simulink library "sm_boom_lift_crawler_lib"  (R2026a)
settings: Solver=VariableStepAuto
undefined symbols (not defined in the file): B, b, base_clr_a, base_clr_d, base_clr_e, base_clr_h, base_clr_s, base_h, base_opc, base_rho, base_t, base_w, F, lines, motion, overlap_l, valves, X, Y, Z
libraries: nesl_utility x155, fl_lib x72, sm_lib x38, SimscapeFluids_lib x18, $bdroot x2, simulink_extras x1, simulink x1, Custom_Valves x1
(part 4 of 4)

== system sm_boom_lift_crawler_lib/Turret Signal ==
  q : Inport
  Bus Creator : BusCreator  Inputs=3
  PS-Simulink Converter1 : nesl_utility/PS-Simulink Converter  PhysicalDomain=network_engine_domain  SubClassName=ps_output  LeftPortType=input  RightPortType=output  PseudoPeriodic=off  Frequencies=[]  VectorFormat=1-D array  Unit=inherit  AffineConversion=off
  PS-Simulink Converter2 : nesl_utility/PS-Simulink Converter  PhysicalDomain=network_engine_domain  SubClassName=ps_output  LeftPortType=input  RightPortType=output  PseudoPeriodic=off  Frequencies=[]  VectorFormat=1-D array  Unit=inherit  AffineConversion=off
  PS-Simulink Converter3 : nesl_utility/PS-Simulink Converter  PhysicalDomain=network_engine_domain  SubClassName=ps_output  LeftPortType=input  RightPortType=output  PseudoPeriodic=off  Frequencies=[]  VectorFormat=1-D array  Unit=inherit  AffineConversion=off
  Revolute Turret : sm_lib/Joints/Revolute Joint  JointMode=Normal  CompositeWrenchDir=FollowerOnBase  CompositeWrenchFrame=BaseFrame  SenseConstraintForce=off  SenseConstraintTorque=off  SenseTotalForce=off  SenseTotalTorque=off  PositionTargetSpecify=on  PositionTargetPriority=High  PositionTargetValue=0  PositionTargetValueUnits=deg  VelocityTargetSpecify=off  VelocityTargetPriority=High  VelocityTargetValue=0  VelocityTargetValueUnits=deg/s  EquilibriumPosition=0  EquilibriumPositionUnits=rad  SpringStiffness=0  SpringStiffnessUnits=N*m/rad  DampingCoefficient=b.r.joint  DampingCoefficientUnits=N*m/(rad/s)  LowerLimitSpecify=off  LowerLimitBound=-90  LowerLimitBoundUnits=deg  LowerLimitStiffness=1e4  LowerLimitStiffnessUnits=N*m/deg  LowerLimitDamping=10  LowerLimitDampingUnits=N*m/(deg/s)  LowerLimitTransitionRegionWidth=0.1  LowerLimitTransitionRegionWidthUnits=deg  UpperLimitSpecify=off  UpperLimitBound=90  UpperLimitBoundUnits=deg  UpperLimitStiffness=1e4  UpperLimitStiffnessUnits=N*m/deg  UpperLimitDamping=10  UpperLimitDampingUnits=N*m/(deg/s)  UpperLimitTransitionRegionWidth=0.1  UpperLimitTransitionRegionWidthUnits=deg  TorqueActuationMode=ComputedTorque  MotionActuationMode=InputMotion  SensePosition=on  SenseVelocity=on  SenseAcceleration=off  SenseTorqueForce=on  SenseLowerLimitTorqueForce=off  SenseUpperLimitTorqueForce=off
  Simscape Bus3 : SimscapeBus  HierarchyStrings=B;F
  Simulink-PS Converter : nesl_utility/Simulink-PS Converter  PhysicalDomain=network_engine_domain  SubClassName=ps_input  LeftPortType=input  RightPortType=output  PseudoPeriodic=off  Frequencies=[]  NoiseDistribution=none  NoiseParameters=[]  Unit=rad  AffineConversion=off  FilteringAndDerivatives=filter  SimscapeFilterOrder=2  InputFilterTimeConstant=0.01  UdotUserProvided=0
  BF : PMIOPort  Side=Right
  m : Outport
  wires:
  PS-Simulink Converter3/1 -> Bus Creator/3  "t"
  Bus Creator/1 -> m/1  "Turret"
  PS-Simulink Converter2/1 -> Bus Creator/2  "w"
  q/1 -> Simulink-PS Converter/1
  PS-Simulink Converter1/1 -> Bus Creator/1  "q"
  connections:
  PS-Simulink Converter3/LConn1 -- Revolute Turret/RConn4
  PS-Simulink Converter2/LConn1 -- Revolute Turret/RConn3
  Simscape Bus3/LConn2 -- Revolute Turret/RConn1
  Simulink-PS Converter/RConn1 -- Revolute Turret/LConn2
  Revolute Turret/RConn2 -- PS-Simulink Converter1/LConn1
  Simscape Bus3/LConn1 -- Revolute Turret/LConn1
  Simscape Bus3/RConn1 -- BF/RConn1

== system sm_boom_lift_crawler_lib/Intf BasketR/Subsystem ==
  PS-Simulink Converter : nesl_utility/PS-Simulink Converter  PhysicalDomain=network_engine_domain  SubClassName=ps_output  LeftPortType=input  RightPortType=output  PseudoPeriodic=off  Frequencies=[]  VectorFormat=1-D array  Unit=inherit  AffineConversion=off
  Simulink-PS Converter : nesl_utility/Simulink-PS Converter  PhysicalDomain=network_engine_domain  SubClassName=ps_input  LeftPortType=input  RightPortType=output  PseudoPeriodic=off  Frequencies=[]  NoiseDistribution=none  NoiseParameters=[]  Unit=N*m  AffineConversion=off  FilteringAndDerivatives=provide  SimscapeFilterOrder=1  InputFilterTimeConstant=0.001  UdotUserProvided=0
  I : PMIOPort  Side=Left
  O : PMIOPort  Port=2  Side=Right
  wires:
  PS-Simulink Converter/1 -> Simulink-PS Converter/1
  connections:
  Simulink-PS Converter/RConn1 -- O/RConn1
  PS-Simulink Converter/LConn1 -- I/RConn1

== system sm_boom_lift_crawler_lib/Intf BasketR/Subsystem1 ==
  PS-Simulink Converter : nesl_utility/PS-Simulink Converter  PhysicalDomain=network_engine_domain  SubClassName=ps_output  LeftPortType=input  RightPortType=output  PseudoPeriodic=off  Frequencies=[]  VectorFormat=1-D array  Unit=inherit  AffineConversion=off
  Simulink-PS Converter : nesl_utility/Simulink-PS Converter  PhysicalDomain=network_engine_domain  SubClassName=ps_input  LeftPortType=input  RightPortType=output  PseudoPeriodic=off  Frequencies=[]  NoiseDistribution=none  NoiseParameters=[]  Unit=rad/s  AffineConversion=off  FilteringAndDerivatives=provide  SimscapeFilterOrder=1  InputFilterTimeConstant=0.001  UdotUserProvided=0
  I : PMIOPort  Side=Left
  O : PMIOPort  Port=2  Side=Right
  wires:
  PS-Simulink Converter/1 -> Simulink-PS Converter/1
  connections:
  PS-Simulink Converter/LConn1 -- I/RConn1
  Simulink-PS Converter/RConn1 -- O/RConn1

== system sm_boom_lift_crawler_lib/Intf Extend/Subsystem ==
  PS-Simulink Converter : nesl_utility/PS-Simulink Converter  PhysicalDomain=network_engine_domain  SubClassName=ps_output  LeftPortType=input  RightPortType=output  PseudoPeriodic=off  Frequencies=[]  VectorFormat=1-D array  Unit=inherit  AffineConversion=off
  Simulink-PS Converter : nesl_utility/Simulink-PS Converter  PhysicalDomain=network_engine_domain  SubClassName=ps_input  LeftPortType=input  RightPortType=output  PseudoPeriodic=off  Frequencies=[]  NoiseDistribution=none  NoiseParameters=[]  Unit=N  AffineConversion=off  FilteringAndDerivatives=provide  SimscapeFilterOrder=1  InputFilterTimeConstant=0.001  UdotUserProvided=0
  I : PMIOPort  Side=Left
  O : PMIOPort  Port=2  Side=Right
  wires:
  PS-Simulink Converter/1 -> Simulink-PS Converter/1
  connections:
  Simulink-PS Converter/RConn1 -- O/RConn1
  PS-Simulink Converter/LConn1 -- I/RConn1

== system sm_boom_lift_crawler_lib/Intf Extend/Subsystem1 ==
  PS-Simulink Converter : nesl_utility/PS-Simulink Converter  PhysicalDomain=network_engine_domain  SubClassName=ps_output  LeftPortType=input  RightPortType=output  PseudoPeriodic=off  Frequencies=[]  VectorFormat=1-D array  Unit=inherit  AffineConversion=off
  Simulink-PS Converter : nesl_utility/Simulink-PS Converter  PhysicalDomain=network_engine_domain  SubClassName=ps_input  LeftPortType=input  RightPortType=output  PseudoPeriodic=off  Frequencies=[]  NoiseDistribution=none  NoiseParameters=[]  Unit=m/s  AffineConversion=off  FilteringAndDerivatives=provide  SimscapeFilterOrder=1  InputFilterTimeConstant=0.001  UdotUserProvided=0
  I : PMIOPort  Side=Left
  O : PMIOPort  Port=2  Side=Right
  wires:
  PS-Simulink Converter/1 -> Simulink-PS Converter/1
  connections:
  PS-Simulink Converter/LConn1 -- I/RConn1
  Simulink-PS Converter/RConn1 -- O/RConn1

== system sm_boom_lift_crawler_lib/Intf Jib/Subsystem ==
  PS-Simulink Converter : nesl_utility/PS-Simulink Converter  PhysicalDomain=network_engine_domain  SubClassName=ps_output  LeftPortType=input  RightPortType=output  PseudoPeriodic=off  Frequencies=[]  VectorFormat=1-D array  Unit=inherit  AffineConversion=off
  Simulink-PS Converter : nesl_utility/Simulink-PS Converter  PhysicalDomain=network_engine_domain  SubClassName=ps_input  LeftPortType=input  RightPortType=output  PseudoPeriodic=off  Frequencies=[]  NoiseDistribution=none  NoiseParameters=[]  Unit=N  AffineConversion=off  FilteringAndDerivatives=provide  SimscapeFilterOrder=1  InputFilterTimeConstant=0.001  UdotUserProvided=0
  I : PMIOPort  Side=Left
  O : PMIOPort  Port=2  Side=Right
  wires:
  PS-Simulink Converter/1 -> Simulink-PS Converter/1
  connections:
  Simulink-PS Converter/RConn1 -- O/RConn1
  PS-Simulink Converter/LConn1 -- I/RConn1

== system sm_boom_lift_crawler_lib/Intf Jib/Subsystem1 ==
  PS-Simulink Converter : nesl_utility/PS-Simulink Converter  PhysicalDomain=network_engine_domain  SubClassName=ps_output  LeftPortType=input  RightPortType=output  PseudoPeriodic=off  Frequencies=[]  VectorFormat=1-D array  Unit=inherit  AffineConversion=off
  Simulink-PS Converter : nesl_utility/Simulink-PS Converter  PhysicalDomain=network_engine_domain  SubClassName=ps_input  LeftPortType=input  RightPortType=output  PseudoPeriodic=off  Frequencies=[]  NoiseDistribution=none  NoiseParameters=[]  Unit=m/s  AffineConversion=off  FilteringAndDerivatives=provide  SimscapeFilterOrder=1  InputFilterTimeConstant=0.001  UdotUserProvided=0
  I : PMIOPort  Side=Left
  O : PMIOPort  Port=2  Side=Right
  wires:
  PS-Simulink Converter/1 -> Simulink-PS Converter/1
  connections:
  PS-Simulink Converter/LConn1 -- I/RConn1
  Simulink-PS Converter/RConn1 -- O/RConn1

== system sm_boom_lift_crawler_lib/Intf Level Master/Subsystem ==
  PS-Simulink Converter : nesl_utility/PS-Simulink Converter  PhysicalDomain=network_engine_domain  SubClassName=ps_output  LeftPortType=input  RightPortType=output  PseudoPeriodic=off  Frequencies=[]  VectorFormat=1-D array  Unit=inherit  AffineConversion=off
  Simulink-PS Converter : nesl_utility/Simulink-PS Converter  PhysicalDomain=network_engine_domain  SubClassName=ps_input  LeftPortType=input  RightPortType=output  PseudoPeriodic=off  Frequencies=[]  NoiseDistribution=none  NoiseParameters=[]  Unit=N  AffineConversion=off  FilteringAndDerivatives=provide  SimscapeFilterOrder=1  InputFilterTimeConstant=0.001  UdotUserProvided=0
  I : PMIOPort  Side=Left
  O : PMIOPort  Port=2  Side=Right
  wires:
  PS-Simulink Converter/1 -> Simulink-PS Converter/1
  connections:
  Simulink-PS Converter/RConn1 -- O/RConn1
  PS-Simulink Converter/LConn1 -- I/RConn1

== system sm_boom_lift_crawler_lib/Intf Level Master/Subsystem1 ==
  PS-Simulink Converter : nesl_utility/PS-Simulink Converter  PhysicalDomain=network_engine_domain  SubClassName=ps_output  LeftPortType=input  RightPortType=output  PseudoPeriodic=off  Frequencies=[]  VectorFormat=1-D array  Unit=inherit  AffineConversion=off
  Simulink-PS Converter : nesl_utility/Simulink-PS Converter  PhysicalDomain=network_engine_domain  SubClassName=ps_input  LeftPortType=input  RightPortType=output  PseudoPeriodic=off  Frequencies=[]  NoiseDistribution=none  NoiseParameters=[]  Unit=m/s  AffineConversion=off  FilteringAndDerivatives=provide  SimscapeFilterOrder=1  InputFilterTimeConstant=0.001  UdotUserProvided=0
  I : PMIOPort  Side=Left
  O : PMIOPort  Port=2  Side=Right
  wires:
  PS-Simulink Converter/1 -> Simulink-PS Converter/1
  connections:
  PS-Simulink Converter/LConn1 -- I/RConn1
  Simulink-PS Converter/RConn1 -- O/RConn1

== system sm_boom_lift_crawler_lib/Intf Level Slave/Subsystem2 ==
  PS-Simulink Converter : nesl_utility/PS-Simulink Converter  PhysicalDomain=network_engine_domain  SubClassName=ps_output  LeftPortType=input  RightPortType=output  PseudoPeriodic=off  Frequencies=[]  VectorFormat=1-D array  Unit=inherit  AffineConversion=off
  Simulink-PS Converter : nesl_utility/Simulink-PS Converter  PhysicalDomain=network_engine_domain  SubClassName=ps_input  LeftPortType=input  RightPortType=output  PseudoPeriodic=off  Frequencies=[]  NoiseDistribution=none  NoiseParameters=[]  Unit=N  AffineConversion=off  FilteringAndDerivatives=provide  SimscapeFilterOrder=1  InputFilterTimeConstant=0.001  UdotUserProvided=0
  I : PMIOPort  Side=Left
  O : PMIOPort  Port=2  Side=Right
  wires:
  PS-Simulink Converter/1 -> Simulink-PS Converter/1
  connections:
  Simulink-PS Converter/RConn1 -- O/RConn1
  PS-Simulink Converter/LConn1 -- I/RConn1

== system sm_boom_lift_crawler_lib/Intf Level Slave/Subsystem3 ==
  PS-Simulink Converter : nesl_utility/PS-Simulink Converter  PhysicalDomain=network_engine_domain  SubClassName=ps_output  LeftPortType=input  RightPortType=output  PseudoPeriodic=off  Frequencies=[]  VectorFormat=1-D array  Unit=inherit  AffineConversion=off
  Simulink-PS Converter : nesl_utility/Simulink-PS Converter  PhysicalDomain=network_engine_domain  SubClassName=ps_input  LeftPortType=input  RightPortType=output  PseudoPeriodic=off  Frequencies=[]  NoiseDistribution=none  NoiseParameters=[]  Unit=m/s  AffineConversion=off  FilteringAndDerivatives=provide  SimscapeFilterOrder=1  InputFilterTimeConstant=0.001  UdotUserProvided=0
  I : PMIOPort  Side=Left
  O : PMIOPort  Port=2  Side=Right
  wires:
  PS-Simulink Converter/1 -> Simulink-PS Converter/1
  connections:
  PS-Simulink Converter/LConn1 -- I/RConn1
  Simulink-PS Converter/RConn1 -- O/RConn1

== system sm_boom_lift_crawler_lib/Intf Lift/Subsystem ==
  PS-Simulink Converter : nesl_utility/PS-Simulink Converter  PhysicalDomain=network_engine_domain  SubClassName=ps_output  LeftPortType=input  RightPortType=output  PseudoPeriodic=off  Frequencies=[]  VectorFormat=1-D array  Unit=inherit  AffineConversion=off
  Simulink-PS Converter : nesl_utility/Simulink-PS Converter  PhysicalDomain=network_engine_domain  SubClassName=ps_input  LeftPortType=input  RightPortType=output  PseudoPeriodic=off  Frequencies=[]  NoiseDistribution=none  NoiseParameters=[]  Unit=N  AffineConversion=off  FilteringAndDerivatives=provide  SimscapeFilterOrder=1  InputFilterTimeConstant=0.001  UdotUserProvided=0
  I : PMIOPort  Side=Left
  O : PMIOPort  Port=2  Side=Right
  wires:
  PS-Simulink Converter/1 -> Simulink-PS Converter/1
  connections:
  Simulink-PS Converter/RConn1 -- O/RConn1
  PS-Simulink Converter/LConn1 -- I/RConn1

== system sm_boom_lift_crawler_lib/Intf Lift/Subsystem1 ==
  PS-Simulink Converter : nesl_utility/PS-Simulink Converter  PhysicalDomain=network_engine_domain  SubClassName=ps_output  LeftPortType=input  RightPortType=output  PseudoPeriodic=off  Frequencies=[]  VectorFormat=1-D array  Unit=inherit  AffineConversion=off
  Simulink-PS Converter : nesl_utility/Simulink-PS Converter  PhysicalDomain=network_engine_domain  SubClassName=ps_input  LeftPortType=input  RightPortType=output  PseudoPeriodic=off  Frequencies=[]  NoiseDistribution=none  NoiseParameters=[]  Unit=m/s  AffineConversion=off  FilteringAndDerivatives=provide  SimscapeFilterOrder=1  InputFilterTimeConstant=0.001  UdotUserProvided=0
  I : PMIOPort  Side=Left
  O : PMIOPort  Port=2  Side=Right
  wires:
  PS-Simulink Converter/1 -> Simulink-PS Converter/1
  connections:
  PS-Simulink Converter/LConn1 -- I/RConn1
  Simulink-PS Converter/RConn1 -- O/RConn1

== system sm_boom_lift_crawler_lib/Intf OutFL/Subsystem ==
  PS-Simulink Converter : nesl_utility/PS-Simulink Converter  PhysicalDomain=network_engine_domain  SubClassName=ps_output  LeftPortType=input  RightPortType=output  PseudoPeriodic=off  Frequencies=[]  VectorFormat=1-D array  Unit=inherit  AffineConversion=off
  Simulink-PS Converter : nesl_utility/Simulink-PS Converter  PhysicalDomain=network_engine_domain  SubClassName=ps_input  LeftPortType=input  RightPortType=output  PseudoPeriodic=off  Frequencies=[]  NoiseDistribution=none  NoiseParameters=[]  Unit=N  AffineConversion=off  FilteringAndDerivatives=provide  SimscapeFilterOrder=1  InputFilterTimeConstant=0.001  UdotUserProvided=0
  I : PMIOPort  Side=Left
  O : PMIOPort  Port=2  Side=Right
  wires:
  PS-Simulink Converter/1 -> Simulink-PS Converter/1
  connections:
  Simulink-PS Converter/RConn1 -- O/RConn1
  PS-Simulink Converter/LConn1 -- I/RConn1

== system sm_boom_lift_crawler_lib/Intf OutFL/Subsystem1 ==
  PS-Simulink Converter : nesl_utility/PS-Simulink Converter  PhysicalDomain=network_engine_domain  SubClassName=ps_output  LeftPortType=input  RightPortType=output  PseudoPeriodic=off  Frequencies=[]  VectorFormat=1-D array  Unit=inherit  AffineConversion=off
  Simulink-PS Converter : nesl_utility/Simulink-PS Converter  PhysicalDomain=network_engine_domain  SubClassName=ps_input  LeftPortType=input  RightPortType=output  PseudoPeriodic=off  Frequencies=[]  NoiseDistribution=none  NoiseParameters=[]  Unit=m/s  AffineConversion=off  FilteringAndDerivatives=provide  SimscapeFilterOrder=1  InputFilterTimeConstant=0.001  UdotUserProvided=0
  I : PMIOPort  Side=Left
  O : PMIOPort  Port=2  Side=Right
  wires:
  PS-Simulink Converter/1 -> Simulink-PS Converter/1
  connections:
  PS-Simulink Converter/LConn1 -- I/RConn1
  Simulink-PS Converter/RConn1 -- O/RConn1

== system sm_boom_lift_crawler_lib/Intf OutFR/Subsystem ==
  PS-Simulink Converter : nesl_utility/PS-Simulink Converter  PhysicalDomain=network_engine_domain  SubClassName=ps_output  LeftPortType=input  RightPortType=output  PseudoPeriodic=off  Frequencies=[]  VectorFormat=1-D array  Unit=inherit  AffineConversion=off
  Simulink-PS Converter : nesl_utility/Simulink-PS Converter  PhysicalDomain=network_engine_domain  SubClassName=ps_input  LeftPortType=input  RightPortType=output  PseudoPeriodic=off  Frequencies=[]  NoiseDistribution=none  NoiseParameters=[]  Unit=N  AffineConversion=off  FilteringAndDerivatives=provide  SimscapeFilterOrder=1  InputFilterTimeConstant=0.001  UdotUserProvided=0
  I : PMIOPort  Side=Left
  O : PMIOPort  Port=2  Side=Right
  wires:
  PS-Simulink Converter/1 -> Simulink-PS Converter/1
  connections:
  Simulink-PS Converter/RConn1 -- O/RConn1
  PS-Simulink Converter/LConn1 -- I/RConn1

== system sm_boom_lift_crawler_lib/Intf OutFR/Subsystem1 ==
  PS-Simulink Converter : nesl_utility/PS-Simulink Converter  PhysicalDomain=network_engine_domain  SubClassName=ps_output  LeftPortType=input  RightPortType=output  PseudoPeriodic=off  Frequencies=[]  VectorFormat=1-D array  Unit=inherit  AffineConversion=off
  Simulink-PS Converter : nesl_utility/Simulink-PS Converter  PhysicalDomain=network_engine_domain  SubClassName=ps_input  LeftPortType=input  RightPortType=output  PseudoPeriodic=off  Frequencies=[]  NoiseDistribution=none  NoiseParameters=[]  Unit=m/s  AffineConversion=off  FilteringAndDerivatives=provide  SimscapeFilterOrder=1  InputFilterTimeConstant=0.001  UdotUserProvided=0
  I : PMIOPort  Side=Left
  O : PMIOPort  Port=2  Side=Right
  wires:
  PS-Simulink Converter/1 -> Simulink-PS Converter/1
  connections:
  PS-Simulink Converter/LConn1 -- I/RConn1
  Simulink-PS Converter/RConn1 -- O/RConn1

== system sm_boom_lift_crawler_lib/Intf OutRL/Subsystem ==
  PS-Simulink Converter : nesl_utility/PS-Simulink Converter  PhysicalDomain=network_engine_domain  SubClassName=ps_output  LeftPortType=input  RightPortType=output  PseudoPeriodic=off  Frequencies=[]  VectorFormat=1-D array  Unit=inherit  AffineConversion=off
  Simulink-PS Converter : nesl_utility/Simulink-PS Converter  PhysicalDomain=network_engine_domain  SubClassName=ps_input  LeftPortType=input  RightPortType=output  PseudoPeriodic=off  Frequencies=[]  NoiseDistribution=none  NoiseParameters=[]  Unit=N  AffineConversion=off  FilteringAndDerivatives=provide  SimscapeFilterOrder=1  InputFilterTimeConstant=0.001  UdotUserProvided=0
  I : PMIOPort  Side=Left
  O : PMIOPort  Port=2  Side=Right
  wires:
  PS-Simulink Converter/1 -> Simulink-PS Converter/1
  connections:
  Simulink-PS Converter/RConn1 -- O/RConn1
  PS-Simulink Converter/LConn1 -- I/RConn1

== system sm_boom_lift_crawler_lib/Intf OutRL/Subsystem1 ==
  PS-Simulink Converter : nesl_utility/PS-Simulink Converter  PhysicalDomain=network_engine_domain  SubClassName=ps_output  LeftPortType=input  RightPortType=output  PseudoPeriodic=off  Frequencies=[]  VectorFormat=1-D array  Unit=inherit  AffineConversion=off
  Simulink-PS Converter : nesl_utility/Simulink-PS Converter  PhysicalDomain=network_engine_domain  SubClassName=ps_input  LeftPortType=input  RightPortType=output  PseudoPeriodic=off  Frequencies=[]  NoiseDistribution=none  NoiseParameters=[]  Unit=m/s  AffineConversion=off  FilteringAndDerivatives=provide  SimscapeFilterOrder=1  InputFilterTimeConstant=0.001  UdotUserProvided=0
  I : PMIOPort  Side=Left
  O : PMIOPort  Port=2  Side=Right
  wires:
  PS-Simulink Converter/1 -> Simulink-PS Converter/1
  connections:
  PS-Simulink Converter/LConn1 -- I/RConn1
  Simulink-PS Converter/RConn1 -- O/RConn1

== system sm_boom_lift_crawler_lib/Intf OutRR/Subsystem ==
  PS-Simulink Converter : nesl_utility/PS-Simulink Converter  PhysicalDomain=network_engine_domain  SubClassName=ps_output  LeftPortType=input  RightPortType=output  PseudoPeriodic=off  Frequencies=[]  VectorFormat=1-D array  Unit=inherit  AffineConversion=off
  Simulink-PS Converter : nesl_utility/Simulink-PS Converter  PhysicalDomain=network_engine_domain  SubClassName=ps_input  LeftPortType=input  RightPortType=output  PseudoPeriodic=off  Frequencies=[]  NoiseDistribution=none  NoiseParameters=[]  Unit=N  AffineConversion=off  FilteringAndDerivatives=provide  SimscapeFilterOrder=1  InputFilterTimeConstant=0.001  UdotUserProvided=0
  I : PMIOPort  Side=Left
  O : PMIOPort  Port=2  Side=Right
  wires:
  PS-Simulink Converter/1 -> Simulink-PS Converter/1
  connections:
  Simulink-PS Converter/RConn1 -- O/RConn1
  PS-Simulink Converter/LConn1 -- I/RConn1

== system sm_boom_lift_crawler_lib/Intf OutRR/Subsystem1 ==
  PS-Simulink Converter : nesl_utility/PS-Simulink Converter  PhysicalDomain=network_engine_domain  SubClassName=ps_output  LeftPortType=input  RightPortType=output  PseudoPeriodic=off  Frequencies=[]  VectorFormat=1-D array  Unit=inherit  AffineConversion=off
  Simulink-PS Converter : nesl_utility/Simulink-PS Converter  PhysicalDomain=network_engine_domain  SubClassName=ps_input  LeftPortType=input  RightPortType=output  PseudoPeriodic=off  Frequencies=[]  NoiseDistribution=none  NoiseParameters=[]  Unit=m/s  AffineConversion=off  FilteringAndDerivatives=provide  SimscapeFilterOrder=1  InputFilterTimeConstant=0.001  UdotUserProvided=0
  I : PMIOPort  Side=Left
  O : PMIOPort  Port=2  Side=Right
  wires:
  PS-Simulink Converter/1 -> Simulink-PS Converter/1
  connections:
  PS-Simulink Converter/LConn1 -- I/RConn1
  Simulink-PS Converter/RConn1 -- O/RConn1

== system sm_boom_lift_crawler_lib/Intf Tilt/Subsystem ==
  PS-Simulink Converter : nesl_utility/PS-Simulink Converter  PhysicalDomain=network_engine_domain  SubClassName=ps_output  LeftPortType=input  RightPortType=output  PseudoPeriodic=off  Frequencies=[]  VectorFormat=1-D array  Unit=inherit  AffineConversion=off
  Simulink-PS Converter : nesl_utility/Simulink-PS Converter  PhysicalDomain=network_engine_domain  SubClassName=ps_input  LeftPortType=input  RightPortType=output  PseudoPeriodic=off  Frequencies=[]  NoiseDistribution=none  NoiseParameters=[]  Unit=N  AffineConversion=off  FilteringAndDerivatives=provide  SimscapeFilterOrder=1  InputFilterTimeConstant=0.001  UdotUserProvided=0
  I : PMIOPort  Side=Left
  O : PMIOPort  Port=2  Side=Right
  wires:
  PS-Simulink Converter/1 -> Simulink-PS Converter/1
  connections:
  Simulink-PS Converter/RConn1 -- O/RConn1
  PS-Simulink Converter/LConn1 -- I/RConn1

== system sm_boom_lift_crawler_lib/Intf Tilt/Subsystem1 ==
  PS-Simulink Converter : nesl_utility/PS-Simulink Converter  PhysicalDomain=network_engine_domain  SubClassName=ps_output  LeftPortType=input  RightPortType=output  PseudoPeriodic=off  Frequencies=[]  VectorFormat=1-D array  Unit=inherit  AffineConversion=off
  Simulink-PS Converter : nesl_utility/Simulink-PS Converter  PhysicalDomain=network_engine_domain  SubClassName=ps_input  LeftPortType=input  RightPortType=output  PseudoPeriodic=off  Frequencies=[]  NoiseDistribution=none  NoiseParameters=[]  Unit=m/s  AffineConversion=off  FilteringAndDerivatives=provide  SimscapeFilterOrder=1  InputFilterTimeConstant=0.001  UdotUserProvided=0
  I : PMIOPort  Side=Left
  O : PMIOPort  Port=2  Side=Right
  wires:
  PS-Simulink Converter/1 -> Simulink-PS Converter/1
  connections:
  PS-Simulink Converter/LConn1 -- I/RConn1
  Simulink-PS Converter/RConn1 -- O/RConn1

== system sm_boom_lift_crawler_lib/Intf TrackL/Subsystem ==
  PS-Simulink Converter : nesl_utility/PS-Simulink Converter  PhysicalDomain=network_engine_domain  SubClassName=ps_output  LeftPortType=input  RightPortType=output  PseudoPeriodic=off  Frequencies=[]  VectorFormat=1-D array  Unit=inherit  AffineConversion=off
  Simulink-PS Converter : nesl_utility/Simulink-PS Converter  PhysicalDomain=network_engine_domain  SubClassName=ps_input  LeftPortType=input  RightPortType=output  PseudoPeriodic=off  Frequencies=[]  NoiseDistribution=none  NoiseParameters=[]  Unit=N  AffineConversion=off  FilteringAndDerivatives=provide  SimscapeFilterOrder=1  InputFilterTimeConstant=0.001  UdotUserProvided=0
  I : PMIOPort  Side=Left
  O : PMIOPort  Port=2  Side=Right
  wires:
  PS-Simulink Converter/1 -> Simulink-PS Converter/1
  connections:
  Simulink-PS Converter/RConn1 -- O/RConn1
  PS-Simulink Converter/LConn1 -- I/RConn1

== system sm_boom_lift_crawler_lib/Intf TrackL/Subsystem1 ==
  PS-Simulink Converter : nesl_utility/PS-Simulink Converter  PhysicalDomain=network_engine_domain  SubClassName=ps_output  LeftPortType=input  RightPortType=output  PseudoPeriodic=off  Frequencies=[]  VectorFormat=1-D array  Unit=inherit  AffineConversion=off
  Simulink-PS Converter : nesl_utility/Simulink-PS Converter  PhysicalDomain=network_engine_domain  SubClassName=ps_input  LeftPortType=input  RightPortType=output  PseudoPeriodic=off  Frequencies=[]  NoiseDistribution=none  NoiseParameters=[]  Unit=m/s  AffineConversion=off  FilteringAndDerivatives=provide  SimscapeFilterOrder=1  InputFilterTimeConstant=0.001  UdotUserProvided=0
  I : PMIOPort  Side=Left
  O : PMIOPort  Port=2  Side=Right
  wires:
  PS-Simulink Converter/1 -> Simulink-PS Converter/1
  connections:
  PS-Simulink Converter/LConn1 -- I/RConn1
  Simulink-PS Converter/RConn1 -- O/RConn1

== system sm_boom_lift_crawler_lib/Intf TrackR/Subsystem2 ==
  PS-Simulink Converter : nesl_utility/PS-Simulink Converter  PhysicalDomain=network_engine_domain  SubClassName=ps_output  LeftPortType=input  RightPortType=output  PseudoPeriodic=off  Frequencies=[]  VectorFormat=1-D array  Unit=inherit  AffineConversion=off
  Simulink-PS Converter : nesl_utility/Simulink-PS Converter  PhysicalDomain=network_engine_domain  SubClassName=ps_input  LeftPortType=input  RightPortType=output  PseudoPeriodic=off  Frequencies=[]  NoiseDistribution=none  NoiseParameters=[]  Unit=N  AffineConversion=off  FilteringAndDerivatives=provide  SimscapeFilterOrder=1  InputFilterTimeConstant=0.001  UdotUserProvided=0
  I : PMIOPort  Side=Left
  O : PMIOPort  Port=2  Side=Right
  wires:
  PS-Simulink Converter/1 -> Simulink-PS Converter/1
  connections:
  Simulink-PS Converter/RConn1 -- O/RConn1
  PS-Simulink Converter/LConn1 -- I/RConn1

== system sm_boom_lift_crawler_lib/Intf TrackR/Subsystem3 ==
  PS-Simulink Converter : nesl_utility/PS-Simulink Converter  PhysicalDomain=network_engine_domain  SubClassName=ps_output  LeftPortType=input  RightPortType=output  PseudoPeriodic=off  Frequencies=[]  VectorFormat=1-D array  Unit=inherit  AffineConversion=off
  Simulink-PS Converter : nesl_utility/Simulink-PS Converter  PhysicalDomain=network_engine_domain  SubClassName=ps_input  LeftPortType=input  RightPortType=output  PseudoPeriodic=off  Frequencies=[]  NoiseDistribution=none  NoiseParameters=[]  Unit=m/s  AffineConversion=off  FilteringAndDerivatives=provide  SimscapeFilterOrder=1  InputFilterTimeConstant=0.001  UdotUserProvided=0
  I : PMIOPort  Side=Left
  O : PMIOPort  Port=2  Side=Right
  wires:
  PS-Simulink Converter/1 -> Simulink-PS Converter/1
  connections:
  PS-Simulink Converter/LConn1 -- I/RConn1
  Simulink-PS Converter/RConn1 -- O/RConn1

== system sm_boom_lift_crawler_lib/Intf Turret/Subsystem ==
  PS-Simulink Converter : nesl_utility/PS-Simulink Converter  PhysicalDomain=network_engine_domain  SubClassName=ps_output  LeftPortType=input  RightPortType=output  PseudoPeriodic=off  Frequencies=[]  VectorFormat=1-D array  Unit=inherit  AffineConversion=off
  Simulink-PS Converter : nesl_utility/Simulink-PS Converter  PhysicalDomain=network_engine_domain  SubClassName=ps_input  LeftPortType=input  RightPortType=output  PseudoPeriodic=off  Frequencies=[]  NoiseDistribution=none  NoiseParameters=[]  Unit=N*m  AffineConversion=off  FilteringAndDerivatives=provide  SimscapeFilterOrder=1  InputFilterTimeConstant=0.001  UdotUserProvided=0
  I : PMIOPort  Side=Left
  O : PMIOPort  Port=2  Side=Right
  wires:
  PS-Simulink Converter/1 -> Simulink-PS Converter/1
  connections:
  Simulink-PS Converter/RConn1 -- O/RConn1
  PS-Simulink Converter/LConn1 -- I/RConn1

== system sm_boom_lift_crawler_lib/Intf Turret/Subsystem1 ==
  PS-Simulink Converter : nesl_utility/PS-Simulink Converter  PhysicalDomain=network_engine_domain  SubClassName=ps_output  LeftPortType=input  RightPortType=output  PseudoPeriodic=off  Frequencies=[]  VectorFormat=1-D array  Unit=inherit  AffineConversion=off
  Simulink-PS Converter : nesl_utility/Simulink-PS Converter  PhysicalDomain=network_engine_domain  SubClassName=ps_input  LeftPortType=input  RightPortType=output  PseudoPeriodic=off  Frequencies=[]  NoiseDistribution=none  NoiseParameters=[]  Unit=rad/s  AffineConversion=off  FilteringAndDerivatives=provide  SimscapeFilterOrder=1  InputFilterTimeConstant=0.001  UdotUserProvided=0
  I : PMIOPort  Side=Left
  O : PMIOPort  Port=2  Side=Right
  wires:
  PS-Simulink Converter/1 -> Simulink-PS Converter/1
  connections:
  PS-Simulink Converter/LConn1 -- I/RConn1
  Simulink-PS Converter/RConn1 -- O/RConn1

== system sm_boom_lift_crawler_lib/Level Slave Signal/Masterp to Slavep ==
  Mp : Inport
  Bias : Bias  Bias=-motion.master.p(1)  SaturateOnIntegerOverflow=off
  Bias1 : Bias  Bias=motion.slave.p(1)  SaturateOnIntegerOverflow=off
  Transfer Fcn (with initial outputs) : simulink_extras/Additional Linear/Transfer Fcn (with initial outputs)  N=[-1.3857]  D="[0.05  1]"  Y0=0  U0=0
  Sp : Outport
  wires:
  Mp/1 -> Bias/1
  Bias/1 -> Transfer Fcn (with initial outputs)/1
  Transfer Fcn (with initial outputs)/1 -> Bias1/1
  Bias1/1 -> Sp/1

== system sm_boom_lift_crawler_lib/Outrigger Actuator/Lower Limit ==
  Min Spool Displacement : fl_lib/Physical Signals/Sources/PS Constant  constant=1.1e-9 m
  PS Add : fl_lib/Physical Signals/Functions/PS Add
  SLim : PMIOPort  Side=Left
  S : PMIOPort  Port=2  Side=Right
  connections:
  Min Spool Displacement/RConn1 -- PS Add/LConn2
  PS Add/RConn1 -- SLim/RConn1
  PS Add/LConn1 -- S/RConn1

== system sm_boom_lift_crawler_lib/Sensor PQ/Flow Rate Sensor ==
  Flow Rate Sensor : fl_lib/Isothermal Liquid/Sensors/Flow Rate Sensor (IL)  sensor_type=3
  V : PMIOPort  Side=Right
  A : PMIOPort  Port=2  Side=Left
  B : PMIOPort  Port=3  Side=Right
  M : PMIOPort  Port=4  Side=Right
  connections:
  A/RConn1 -- Flow Rate Sensor/LConn1
  Flow Rate Sensor/RConn2 -- M/RConn1
  Flow Rate Sensor/RConn1 -- B/RConn1
  Flow Rate Sensor/RConn3 -- V/RConn1

== system sm_boom_lift_crawler_lib/Sensor PQ AB/Flow Rate Sensor ==
  Flow Rate Sensor : fl_lib/Isothermal Liquid/Sensors/Flow Rate Sensor (IL)  sensor_type=3
  V : PMIOPort  Side=Right
  A : PMIOPort  Port=2  Side=Left
  B : PMIOPort  Port=3  Side=Right
  M : PMIOPort  Port=4  Side=Right
  connections:
  A/RConn1 -- Flow Rate Sensor/LConn1
  Flow Rate Sensor/RConn2 -- M/RConn1
  Flow Rate Sensor/RConn1 -- B/RConn1
  Flow Rate Sensor/RConn3 -- V/RConn1
